simulink model "ProbotISCI2016"  (Simulink 8.4)
settings: Solver=ode45  StartTime=0.0  StopTime=100  RelTol=1e-3
libraries: fuzblock x1
settings Model: Creator=Ricardo Martinez  LastModifiedBy=oscar  ExtModeTrigMode=oneshot  ExtModeArmWhenConnect=off  BufferReuse=off
settings SolverCC: ZeroCrossControl=DisableAll
settings DataIOCC: LimitDataPoints=off
settings OptimizationCC: BlockReduction=off  BooleanDataType=off  OptimizeBlockIOStorage=off  BufferReuse=off  GlobalBufferReuse=off  ExpressionFolding=off  LocalBlockOutputs=off  InitFltsAndDblsToZero=on
settings DebuggingCC: SaveWithParameterizedLinksMsg=none  SignalResolutionControl=TryResolveAllWithWarning  SolverPrmCheckMsg=none  MultiTaskDSMMsg=warning  MultiTaskCondExecSysMsg=none  FrameProcessingCompatibilityMsg=error
settings HardwareCC: TargetBitPerLong=64  TargetBitPerPointer=64  TargetLongLongMode=on  TargetIntDivRoundTo=Zero  TargetEndianess=LittleEndian  TargetWordSize=64  TargetHWDeviceType=MATLAB Host  ProdEqTarget=off
settings GRTTargetCC: TargetFcnLib=ansi_tfl_tmw.mat
settings ConfigComp: CovMetricSettings=dw  CovHtmlReporting=on  CovSaveCumulativeToWorkspaceVar=on  CovSaveSingleToWorkspaceVar=on  CovModelRefEnable=Off  CovExternalEMLEnable=off

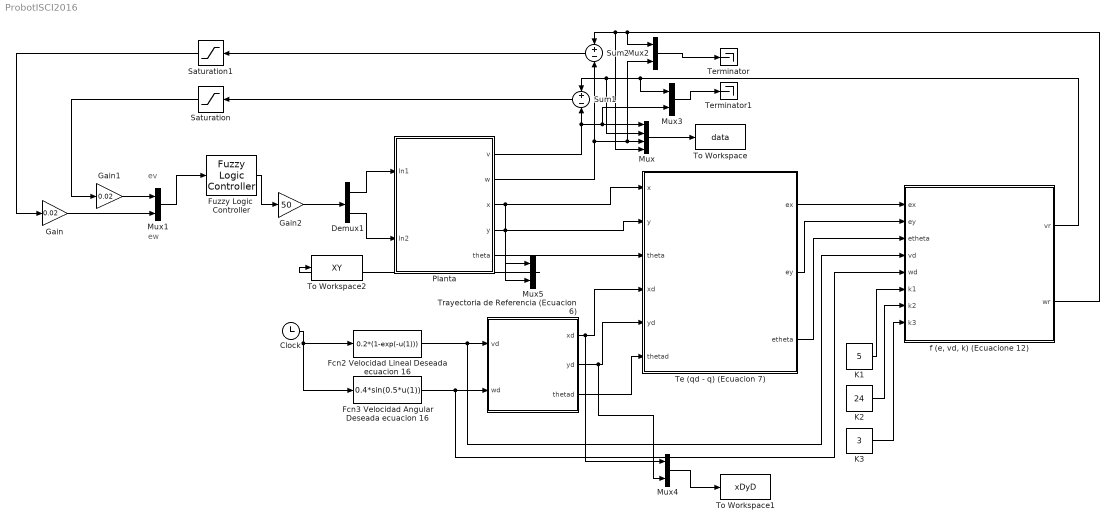
== system ProbotISCI2016 ==
  note: ev
  note: ew
  Clock : Clock
      settings: Decimation=200
  Demux1 : Demux  Outputs=2
  Fcn2 Velocidad Lineal Deseada ecuacion 16 : Fcn  Expr=0.2*(1-exp(-u(1)))
  Fcn3 Velocidad Angular Deseada ecuacion 16 : Fcn  Expr=0.4*sin(0.5*u(1))
  Fuzzy Logic  Controller : fuzblock/Fuzzy Logic  Controller  fis='BaseRobotFA.fis'
  Gain : Gain  Gain=0.02
  Gain1 : Gain  Gain=0.02
  Gain2 : Gain  Gain=50
  K1 : Constant  Value=5
  K2 : Constant  Value=24
  K3 : Constant  Value=3
  Mux : Mux
  Mux{1..5} (5 alike) : Mux  Inputs=2
  Planta : Subsystem
  Saturation : Saturate  UpperLimit=50  LowerLimit=-50
  Saturation1 : Saturate  UpperLimit=50  LowerLimit=-50
  Sum1 : Sum  Inputs=+-  SaturateOnIntegerOverflow=on  InputSameDT=on  OutDataTypeStr=Inherit: Same as first input
  Sum2 : Sum  Inputs=+-  SaturateOnIntegerOverflow=on  InputSameDT=on  OutDataTypeStr=Inherit: Same as first input
  Te (qd - q) (Ecuacion 7) : Subsystem
  Terminator : Terminator
  Terminator1 : Terminator
  To Workspace : ToWorkspace  VariableName=data  SaveFormat=Structure  SampleTime=-1
      settings: MaxDataPoints=80
  To Workspace1 : ToWorkspace  VariableName=xDyD  SaveFormat=Structure  SampleTime=-1
  To Workspace2 : ToWorkspace  VariableName=XY  SaveFormat=Structure  SampleTime=-1
  Trayectoria de Referencia (Ecuacion 6) : Subsystem
  "f (e, vd, k) (Ecuacione 12)" : Subsystem
  wires:
  Trayectoria de Referencia (Ecuacion 6)/1(xd) -> Te (qd - q) (Ecuacion 7)/4(xd), Mux4/1
  Trayectoria de Referencia (Ecuacion 6)/3(thetad) -> Te (qd - q) (Ecuacion 7)/6(thetad)
  Trayectoria de Referencia (Ecuacion 6)/2(yd) -> Te (qd - q) (Ecuacion 7)/5(yd), Mux4/2
  Te (qd - q) (Ecuacion 7)/1(ex) -> "f (e, vd, k) (Ecuacione 12)"/1(ex)
  Te (qd - q) (Ecuacion 7)/2(ey) -> "f (e, vd, k) (Ecuacione 12)"/2(ey)
  Te (qd - q) (Ecuacion 7)/3(etheta) -> "f (e, vd, k) (Ecuacione 12)"/3(etheta)
  Fcn2 Velocidad Lineal Deseada ecuacion 16/1 -> Trayectoria de Referencia (Ecuacion 6)/1(vd), "f (e, vd, k) (Ecuacione 12)"/4(vd)
  K1/1 -> "f (e, vd, k) (Ecuacione 12)"/6(k1)
  K2/1 -> "f (e, vd, k) (Ecuacione 12)"/7(k2)
  K3/1 -> "f (e, vd, k) (Ecuacione 12)"/8(k3)
  "f (e, vd, k) (Ecuacione 12)"/2(wr) -> Sum2/1, Mux/4, Mux2/1
  "f (e, vd, k) (Ecuacione 12)"/1(vr) -> Sum1/1, Mux/2, Mux3/1
  Planta/5(theta) -> Te (qd - q) (Ecuacion 7)/3(theta)
  Planta/4(y) -> Te (qd - q) (Ecuacion 7)/2(y), Mux5/2
  Planta/3(x) -> Te (qd - q) (Ecuacion 7)/1(x), Mux5/1
  Planta/1(v) -> Sum1/2, Mux/1, Mux3/2
  Fcn3 Velocidad Angular Deseada ecuacion 16/1 -> Trayectoria de Referencia (Ecuacion 6)/2(wd), "f (e, vd, k) (Ecuacione 12)"/5(wd)
  Demux1/1 -> Planta/1(In1)
  Demux1/2 -> Planta/2(In2)
  Clock/1 -> Fcn3 Velocidad Angular Deseada ecuacion 16/1, Fcn2 Velocidad Lineal Deseada ecuacion 16/1
  Planta/2(w) -> Sum2/2, Mux/3, Mux2/2
  Mux/1 -> To Workspace/1
  Sum2/1 -> Saturation1/1
  Fuzzy Logic  Controller/1 -> Gain2/1
  Sum1/1 -> Saturation/1
  Saturation/1 -> Gain1/1
  Saturation1/1 -> Gain/1
  Gain/1 -> Mux1/2
  Gain1/1 -> Mux1/1
  Gain2/1 -> Demux1/1
  Mux4/1 -> To Workspace1/1
  Mux5/1 -> To Workspace2/1
  Mux2/1 -> Terminator/1
  Mux3/1 -> Terminator1/1
  Mux1/1 -> Fuzzy Logic  Controller/1

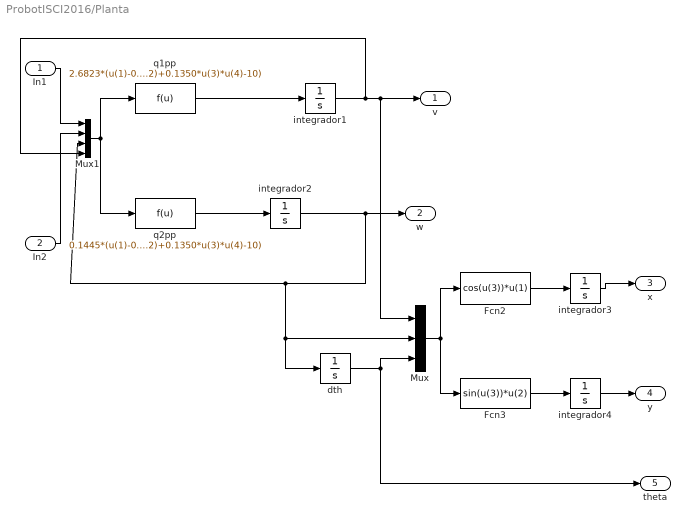
== system ProbotISCI2016/Planta ==
  In1 : Inport
  In2 : Inport  Port=2
  Fcn2 : Fcn  Expr=cos(u(3))*u(1)
  Fcn3 : Fcn  Expr=sin(u(3))*u(2)
  Mux : Mux  Inputs=3
  Mux1 : Mux
  dth : Integrator
  integrador{1..4} (4 alike) : Integrator
  q1pp : Fcn  Expr=2.6823*(u(1)-0.1350*u(3)*u(3)-10)+0.1445*(u(2)+0.1350*u(3)*u(4)-10)
  q2pp : Fcn  Expr=0.1445*(u(1)-0.1350*u(3)*u(3)-10)+2.6823*(u(2)+0.1350*u(3)*u(4)-10)
  v : Outport
  w : Outport  Port=2
  x : Outport  Port=3
  y : Outport  Port=4
  theta : Outport  Port=5
  wires:
  In2/1 -> Mux1/2
  In1/1 -> Mux1/1
  Mux1/1 -> q1pp/1, q2pp/1
  integrador1/1 -> Mux1/4, v/1, Mux/1
  q1pp/1 -> integrador1/1
  q2pp/1 -> integrador2/1
  integrador2/1 -> w/1, Mux1/3, dth/1, Mux/2
  Fcn2/1 -> integrador3/1
  Mux/1 -> Fcn2/1, Fcn3/1
  Fcn3/1 -> integrador4/1
  dth/1 -> theta/1, Mux/3
  integrador3/1 -> x/1
  integrador4/1 -> y/1

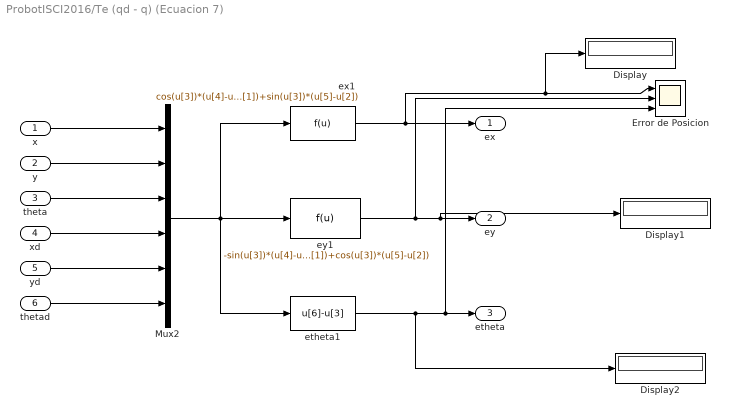
== system ProbotISCI2016/Te (qd - q) (Ecuacion 7) ==
  x : Inport
  y : Inport  Port=2
  theta : Inport  Port=3
  xd : Inport  Port=4
  yd : Inport  Port=5
  thetad : Inport  Port=6
  Display : Display
  Display1 : Display
  Display2 : Display
  Error de Posicion : Scope  NumInputPorts=3
  Mux2 : Mux  Inputs=6
  etheta1 : Fcn  Expr=u[6]-u[3]
  ex1 : Fcn  Expr=cos(u[3])*(u[4]-u[1])+sin(u[3])*(u[5]-u[2])
  ey1 : Fcn  Expr=-sin(u[3])*(u[4]-u[1])+cos(u[3])*(u[5]-u[2])
  ex : Outport
  ey : Outport  Port=2
  etheta : Outport  Port=3
  wires:
  x/1 -> Mux2/1
  y/1 -> Mux2/2
  thetad/1 -> Mux2/6
  Mux2/1 -> ex1/1, etheta1/1, ey1/1
  theta/1 -> Mux2/3
  xd/1 -> Mux2/4
  yd/1 -> Mux2/5
  ex1/1 -> ex/1, Error de Posicion/1, Display/1
  ey1/1 -> Error de Posicion/2, ey/1, Display1/1
  etheta1/1 -> etheta/1, Error de Posicion/3, Display2/1

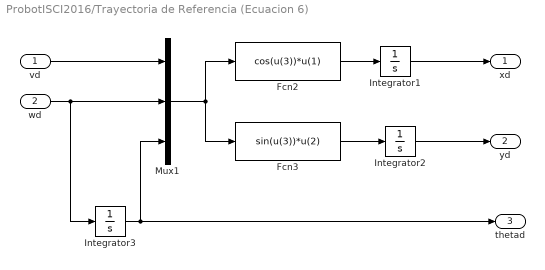
== system ProbotISCI2016/Trayectoria de Referencia (Ecuacion 6) ==
  vd : Inport
  wd : Inport  Port=2
  Fcn2 : Fcn  Expr=cos(u(3))*u(1)
  Fcn3 : Fcn  Expr=sin(u(3))*u(2)
  Integrator1 : Integrator
  Integrator2 : Integrator
  Integrator3 : Integrator
  Mux1 : Mux  Inputs=3
  xd : Outport
  yd : Outport  Port=2
  thetad : Outport  Port=3
  wires:
  Fcn2/1 -> Integrator1/1
  vd/1 -> Mux1/1
  wd/1 -> Mux1/2, Integrator3/1
  Integrator1/1 -> xd/1
  Integrator2/1 -> yd/1
  Fcn3/1 -> Integrator2/1
  Mux1/1 -> Fcn2/1, Fcn3/1
  Integrator3/1 -> Mux1/3, thetad/1

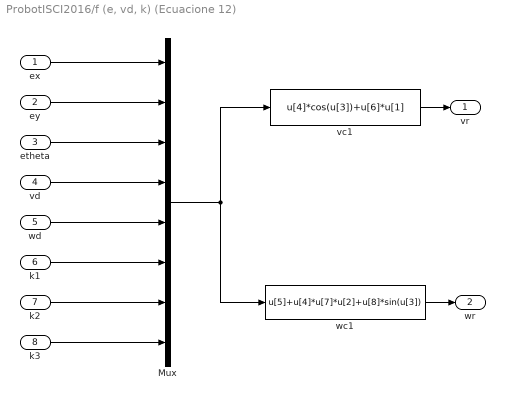
== system ProbotISCI2016/f (e, vd, k) (Ecuacione 12) ==
  ex : Inport
  ey : Inport  Port=2
  etheta : Inport  Port=3
  vd : Inport  Port=4
  wd : Inport  Port=5
  k1 : Inport  Port=6
  k2 : Inport  Port=7
  k3 : Inport  Port=8
  Mux : Mux  Inputs=8
  vc1 : Fcn  Expr=u[4]*cos(u[3])+u[6]*u[1]
  wc1 : Fcn  Expr=u[5]+u[4]*u[7]*u[2]+u[8]*sin(u[3])
  vr : Outport
  wr : Outport  Port=2
  wires:
  vc1/1 -> vr/1
  wc1/1 -> wr/1
  ex/1 -> Mux/1
  ey/1 -> Mux/2
  etheta/1 -> Mux/3
  vd/1 -> Mux/4
  wd/1 -> Mux/5
  k1/1 -> Mux/6
  k2/1 -> Mux/7
  k3/1 -> Mux/8
  Mux/1 -> vc1/1, wc1/1
